simulink model "fsm_for_robot_project"  (R2016a)
settings: Solver=FixedStepDiscrete  StartTime=0.0  StopTime=10.0  FixedStep=0.1  RelTol=1e-3
settings Model: Creator=yettbh  LastModifiedBy=yettbh
settings SolverCC: AutoInsertRateTranBlk=on
settings DataIOCC: LimitDataPoints=on
settings DebuggingCC: AllowSymbolicDim=off
settings ConfigComp: CovModelRefEnable=Off  CovSFcnEnable=off

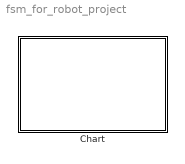
== system fsm_for_robot_project ==
  Chart : Stateflow chart  TreatAsAtomicUnit=on

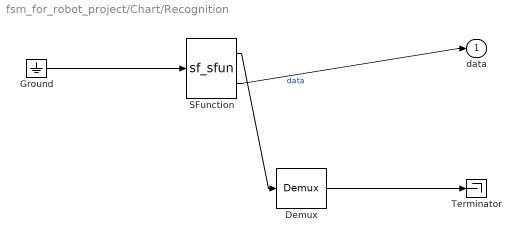
== system fsm_for_robot_project/Chart/Recognition ==
  " Demux " : Demux  Outputs=1
  " Ground " : Ground
  " SFunction " : S-Function  Tag=Stateflow S-Function fsm_for_robot_project 2  FunctionName=sf_sfun  PortCounts=[1 2]  SFunctionDeploymentMode=off  EnableBusSupport=on
  " Terminator " : Terminator
  data : Outport
  wires:
  " SFunction "/2 -> data/1  "data"
  " Ground "/1 -> " SFunction "/1
  " Demux "/1 -> " Terminator "/1
  " SFunction "/1 -> " Demux "/1

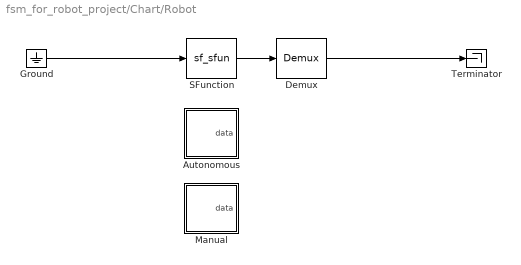
== system fsm_for_robot_project/Chart/Robot ==
  " Demux " : Demux  Outputs=1
  " Ground " : Ground
  " SFunction " : S-Function  Tag=Stateflow S-Function fsm_for_robot_project 1  FunctionName=sf_sfun  PortCounts=[1 1]  SFunctionDeploymentMode=off  EnableBusSupport=off
  " Terminator " : Terminator
  Autonomous : Stateflow chart  TreatAsAtomicUnit=on
      settings: CopyFcn=set_param(gcbh, 'DSMNames', '', 'DSMValues', '', 'CopyFcn', '')
  Manual : Stateflow chart  TreatAsAtomicUnit=on
      settings: CopyFcn=set_param(gcbh, 'DSMNames', '', 'DSMValues', '', 'CopyFcn', '')
  wires:
  " Ground "/1 -> " SFunction "/1
  " Demux "/1 -> " Terminator "/1
  " SFunction "/1 -> " Demux "/1

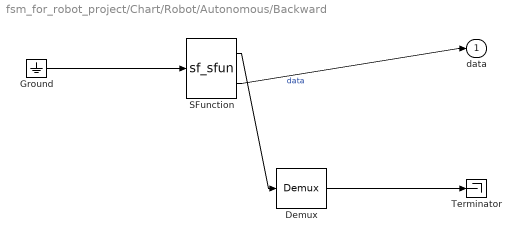
== system fsm_for_robot_project/Chart/Robot/Autonomous/Backward ==
  " Demux " : Demux  Outputs=1
  " Ground " : Ground
  " SFunction " : S-Function  Tag=Stateflow S-Function fsm_for_robot_project 12  FunctionName=sf_sfun  PortCounts=[1 2]  SFunctionDeploymentMode=off  EnableBusSupport=on
  " Terminator " : Terminator
  data : Outport
  wires:
  " SFunction "/2 -> data/1  "data"
  " Ground "/1 -> " SFunction "/1
  " Demux "/1 -> " Terminator "/1
  " SFunction "/1 -> " Demux "/1

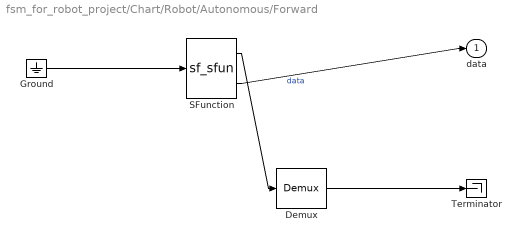
== system fsm_for_robot_project/Chart/Robot/Autonomous/Forward ==
  " Demux " : Demux  Outputs=1
  " Ground " : Ground
  " SFunction " : S-Function  Tag=Stateflow S-Function fsm_for_robot_project 13  FunctionName=sf_sfun  PortCounts=[1 2]  SFunctionDeploymentMode=off  EnableBusSupport=on
  " Terminator " : Terminator
  data : Outport
  wires:
  " SFunction "/2 -> data/1  "data"
  " Ground "/1 -> " SFunction "/1
  " Demux "/1 -> " Terminator "/1
  " SFunction "/1 -> " Demux "/1

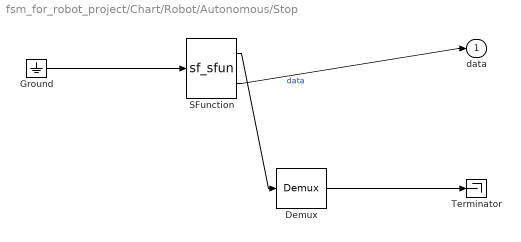
== system fsm_for_robot_project/Chart/Robot/Autonomous/Stop ==
  " Demux " : Demux  Outputs=1
  " Ground " : Ground
  " SFunction " : S-Function  Tag=Stateflow S-Function fsm_for_robot_project 14  FunctionName=sf_sfun  PortCounts=[1 2]  SFunctionDeploymentMode=off  EnableBusSupport=on
  " Terminator " : Terminator
  data : Outport
  wires:
  " SFunction "/2 -> data/1  "data"
  " Ground "/1 -> " SFunction "/1
  " Demux "/1 -> " Terminator "/1
  " SFunction "/1 -> " Demux "/1

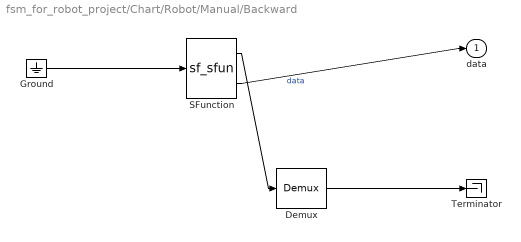
== system fsm_for_robot_project/Chart/Robot/Manual/Backward ==
  " Demux " : Demux  Outputs=1
  " Ground " : Ground
  " SFunction " : S-Function  Tag=Stateflow S-Function fsm_for_robot_project 8  FunctionName=sf_sfun  PortCounts=[1 2]  SFunctionDeploymentMode=off  EnableBusSupport=on
  " Terminator " : Terminator
  data : Outport
  wires:
  " SFunction "/2 -> data/1  "data"
  " Ground "/1 -> " SFunction "/1
  " Demux "/1 -> " Terminator "/1
  " SFunction "/1 -> " Demux "/1

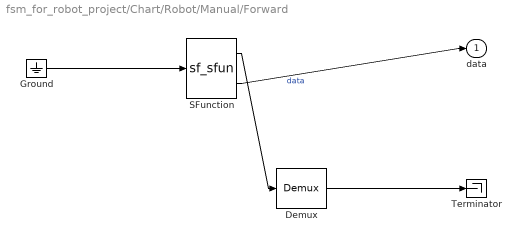
== system fsm_for_robot_project/Chart/Robot/Manual/Forward ==
  " Demux " : Demux  Outputs=1
  " Ground " : Ground
  " SFunction " : S-Function  Tag=Stateflow S-Function fsm_for_robot_project 10  FunctionName=sf_sfun  PortCounts=[1 2]  SFunctionDeploymentMode=off  EnableBusSupport=on
  " Terminator " : Terminator
  data : Outport
  wires:
  " SFunction "/2 -> data/1  "data"
  " Ground "/1 -> " SFunction "/1
  " Demux "/1 -> " Terminator "/1
  " SFunction "/1 -> " Demux "/1

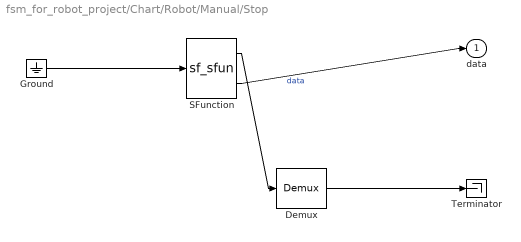
== system fsm_for_robot_project/Chart/Robot/Manual/Stop ==
  " Demux " : Demux  Outputs=1
  " Ground " : Ground
  " SFunction " : S-Function  Tag=Stateflow S-Function fsm_for_robot_project 9  FunctionName=sf_sfun  PortCounts=[1 2]  SFunctionDeploymentMode=off  EnableBusSupport=on
  " Terminator " : Terminator
  data : Outport
  wires:
  " SFunction "/2 -> data/1  "data"
  " Ground "/1 -> " SFunction "/1
  " Demux "/1 -> " Terminator "/1
  " SFunction "/1 -> " Demux "/1

== stateflow chart fsm_for_robot_project/Chart/Robot ==
  state Manual
  state Autonomous
  (default) -> Manual
  Autonomous -> Manual
  Manual -> Autonomous

== stateflow chart fsm_for_robot_project/Chart/Recognition ==
  state Sample Kinect Sensors
  state Process Frame (Sensor Data)
  state Analyze Motion
  (default) -> Sample Kinect Sensors
  Sample Kinect Sensors -> Process Frame (Sensor Data) [order 1] : [frame]
  Sample Kinect Sensors -> Sample Kinect Sensors [order 2] : [~frame]
  Process Frame (Sensor Data) -> Sample Kinect Sensors [order 2] : [frame_count<size]
  Process Frame (Sensor Data) -> Analyze Motion [order 1] : [frame_count>=size]
  Analyze Motion -> Sample Kinect Sensors
  data: data output

== stateflow chart fsm_for_robot_project/Chart ==
  state Recognition Software
  state Robot Controller
  Recognition Software -> Robot Controller

== stateflow chart fsm_for_robot_project/Chart/Robot/Manual ==
  state Stop
  state Backward
  state Forward
  (default) -> Stop [order 1]
  Stop -> Forward
  (default) -> Backward [order 2]
  (default) -> Stop [order 5]
  (default) -> Stop [order 3]
  (default) -> Forward [order 6]
  (default) -> Backward [order 4]
  data: data output

== stateflow chart fsm_for_robot_project/Chart/Robot/Manual/Backward ==
  state Backward
  state TurnL
  state TurnR
  (default) -> Backward
  Backward -> TurnR [order 2]
  Backward -> TurnL [order 1]
  TurnL -> Backward [order 1]
  TurnR -> Backward [order 1]
  TurnL -> TurnR [order 2]
  TurnR -> TurnL [order 2]
  data: data output

== stateflow chart fsm_for_robot_project/Chart/Robot/Manual/Stop ==
  state Stop
  state TurnL
  state TurnR
  (default) -> Stop
  Stop -> TurnR [order 2]
  Stop -> TurnL [order 1]
  TurnL -> Stop [order 1]
  TurnR -> Stop [order 1]
  TurnL -> TurnR [order 2]
  TurnR -> TurnL [order 2]
  data: data output

== stateflow chart fsm_for_robot_project/Chart/Robot/Manual/Forward ==
  state Forward
  state TurnL
  state TurnR
  (default) -> Forward
  Forward -> TurnR [order 2]
  Forward -> TurnL [order 1]
  TurnL -> Forward [order 1]
  TurnR -> Forward [order 1]
  TurnL -> TurnR [order 2]
  TurnR -> TurnL [order 2]
  data: data output

== stateflow chart fsm_for_robot_project/Chart/Robot/Autonomous ==
  state Stop
  state Backward
  state Forward
  (default) -> Stop [order 1]
  Stop -> Forward
  (default) -> Backward [order 2]
  (default) -> Stop [order 5]
  (default) -> Stop [order 3]
  (default) -> Forward [order 6]
  (default) -> Backward [order 4]
  data: data output

== stateflow chart fsm_for_robot_project/Chart/Robot/Autonomous/Backward ==
  state Backward
  state TurnL
  state TurnR
  (default) -> Backward
  Backward -> TurnR [order 2]
  Backward -> TurnL [order 1]
  TurnL -> Backward [order 1]
  TurnR -> Backward [order 1]
  TurnL -> TurnR [order 2]
  TurnR -> TurnL [order 2]
  data: data output

== stateflow chart fsm_for_robot_project/Chart/Robot/Autonomous/Forward ==
  state Forward
  state TurnL
  state TurnR
  (default) -> Forward
  Forward -> TurnR [order 2]
  Forward -> TurnL [order 1]
  TurnL -> Forward [order 1]
  TurnR -> Forward [order 1]
  TurnL -> TurnR [order 2]
  TurnR -> TurnL [order 2]
  data: data output

== stateflow chart fsm_for_robot_project/Chart/Robot/Autonomous/Stop ==
  state Stop
  state TurnL
  state TurnR
  (default) -> Stop
  Stop -> TurnR [order 2]
  Stop -> TurnL [order 1]
  TurnL -> Stop [order 1]
  TurnR -> Stop [order 1]
  TurnL -> TurnR [order 2]
  TurnR -> TurnL [order 2]
  data: data output
